simulink model "Intergration_simu"  (R2018b)
(part 3 of 31)

  SCS_HSC2_FrP24_0x251/5 -> Data Type Conversion71/1  "ChACCAEBBrkJerkReqRespHSC2"
  Data Type Conversion72/1 -> Bus Creator16/4
  SCS_HSC2_FrP24_0x251/6 -> Data Type Conversion72/1  "ChAEBPrflReqRespHSC2"
  Data Type Conversion73/1 -> Bus Creator16/5
  SCS_HSC2_FrP24_0x251/7 -> Data Type Conversion73/1  "ChACCReqFlrStsHSC2"
  Data Type Conversion74/1 -> Bus Creator16/6
  SCS_HSC2_FrP24_0x251/8 -> Data Type Conversion74/1  "ChAEBHydBrkAstReqRespHSC2"
  Data Type Conversion75/1 -> Bus Creator16/7
  SCS_HSC2_FrP24_0x251/9 -> Data Type Conversion75/1  "ChACCAccReqRespHSC2"
  Data Type Conversion76/1 -> Bus Creator16/8
  SCS_HSC2_FrP24_0x251/10 -> Data Type Conversion76/1  "VehSdslStsHSC2"
  Data Type Conversion77/1 -> Bus Creator17/1
  GW_HSC2_HCU_FrP13_0x19C/2 -> Data Type Conversion77/1  "EPTTrInptShaftSpdHSC2"
  Data Type Conversion78/1 -> Bus Creator17/2
  GW_HSC2_HCU_FrP13_0x19C/3 -> Data Type Conversion78/1  "EPTTrInptShaftToqHSC2"
  Data Type Conversion79/1 -> Bus Creator17/3
  GW_HSC2_HCU_FrP13_0x19C/4 -> Data Type Conversion79/1  "EPTTrInptShaftSpdVHSC2"
  Data Type Conversion80/1 -> Bus Creator17/4
  GW_HSC2_HCU_FrP13_0x19C/5 -> Data Type Conversion80/1  "EPTTrInptShaftToqVHSC2"
  Bus Creator17/1 -> Bus Creator9/17
  Bus Creator16/1 -> Bus Creator9/16
  SAS_HSC2_FrP00_0x1E5/8 -> Data Type Conversion13/1  "StrgWhlAngSnsrInidHSC2"
  SAS_HSC2_FrP00_0x1E5/10 -> Data Type Conversion14/1  "StrgWhlAngVHSC2"
  SAS_HSC2_FrP00_0x1E5/9 -> Data Type Conversion26/1  "StrgWhlAngSnsrCalStsHSC2"
  SAS_HSC2_FrP00_0x1E5/6 -> Data Type Conversion11/1  "StrgWhlAngSnsrFltHSC2"
  SAS_HSC2_FrP00_0x1E5/3 -> Data Type Conversion24/1  "StrgWhlAngGrdHSC2"
  SAS_HSC2_FrP00_0x1E5/7 -> Data Type Conversion12/1  "StrgWhlAngSnsrMultCapbHSC2"
  SAS_HSC2_FrP00_0x1E5/5 -> Data Type Conversion25/1  "StrgWhlAngHSC2"
  GW_HSC2_BCM_FrP04_0x46A/18 -> Data Type Conversion62/1  "DircnIndLampSwStsHSC2"
